simulink model "provablock"  (Simulink 7.4)
settings: Solver=ode45  StartTime=0.0  StopTime=10.0  RelTol=1e-3
values from neighbouring files (symbols this model uses):
  robot = wam    [WAMforcecontrol.m]    (also in batchwamobs.m; controltest.m; feedforward.m; inertia2.m = p560)
undefined symbols (not defined in the file or in its folder): selectde, selectdx1e, selectdx2e
settings Model: Creator=acolome  LastModifiedBy=acolome

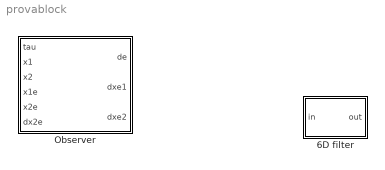
== system provablock ==
  6D filter : Subsystem  mask{K=1, tau=6*pi}
      mask prompts: K "Gain"; tau "time constant"
  Observer : Subsystem  mask{robot=robot, g=[0 0 9.81]}
      mask prompts: robot "Robot Object"; g "Gravity"
      mask Display:
      | port_label('output',1,'de')
      | port_label('output', 2, 'dxe1')
      | port_label('output', 3, 'dxe2')
      | 
      | port_label('input', 1, 'tau')
      | port_label('input', 2, 'q')
      | port_label('input', 3, 'dq')
      | port_label('input', 4, 'x1e')
      | port_label('input', 5, 'x2e')
      | port_label('input', 6, 'dx2e')

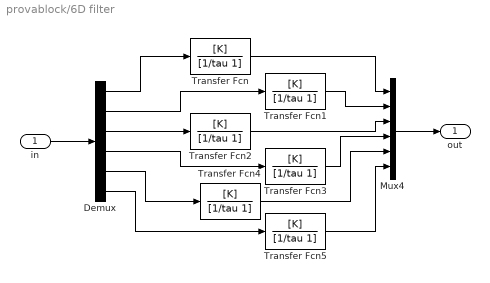
== system provablock/6D filter ==
  in : Inport  OutDataType=fixdt(1, 16)  OutScaling=2^0
  Demux : Demux  Outputs=6
  Mux4 : Mux  Inputs=6
  Transfer Fcn{,1..5} (6 alike) : TransferFcn  Numerator=[K]  Denominator=[1/tau 1]
  out : Outport  OutDataType=fixdt(1, 16)  OutScaling=2^0
  wires:
  Demux/1 -> Transfer Fcn/1
  Demux/2 -> Transfer Fcn1/1
  Demux/3 -> Transfer Fcn2/1
  Demux/4 -> Transfer Fcn3/1
  Demux/5 -> Transfer Fcn4/1
  Demux/6 -> Transfer Fcn5/1
  Transfer Fcn/1 -> Mux4/1
  Transfer Fcn1/1 -> Mux4/2
  Transfer Fcn2/1 -> Mux4/3
  Transfer Fcn3/1 -> Mux4/4
  Transfer Fcn4/1 -> Mux4/5
  Transfer Fcn5/1 -> Mux4/6
  Mux4/1 -> out/1
  in/1 -> Demux/1

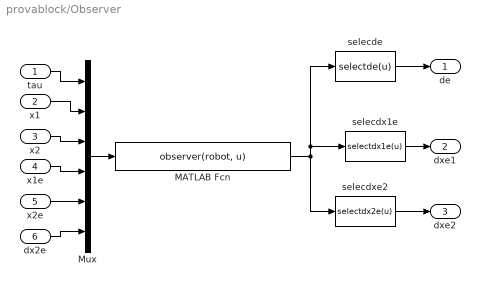
== system provablock/Observer ==
  tau : Inport  OutDataType=fixdt(1, 16)  OutScaling=2^0
  x1 : Inport  Port=2  OutDataType=fixdt(1, 16)  OutScaling=2^0
  x2 : Inport  Port=3  OutDataType=fixdt(1, 16)  OutScaling=2^0
  x1e : Inport  Port=4  OutDataType=fixdt(1, 16)  OutScaling=2^0
  x2e : Inport  Port=5  OutDataType=fixdt(1, 16)  OutScaling=2^0
  dx2e : Inport  Port=6  OutDataType=fixdt(1, 16)  OutScaling=2^0
  MATLAB Fcn : MATLABFcn  MATLABFcn=observer(robot, u)  OutputDimensions=n
  Mux : Mux  Inputs=6
  selecde : MATLABFcn  MATLABFcn=selectde(u)
  selecdx1e : MATLABFcn  MATLABFcn=selectdx1e(u)
  selecdxe2 : MATLABFcn  MATLABFcn=selectdx2e(u)
  de : Outport  OutDataType=fixdt(1, 16)  OutScaling=2^0
  dxe1 : Outport  Port=2  OutDataType=fixdt(1, 16)  OutScaling=2^0
  dxe2 : Outport  Port=3  OutDataType=fixdt(1, 16)  OutScaling=2^0
  wires:
  Mux/1 -> MATLAB Fcn/1
  tau/1 -> Mux/1
  x1/1 -> Mux/2
  x2/1 -> Mux/3
  x1e/1 -> Mux/4
  x2e/1 -> Mux/5
  dx2e/1 -> Mux/6
  MATLAB Fcn/1 -> selecde/1, selecdx1e/1, selecdxe2/1
  selecde/1 -> de/1
  selecdx1e/1 -> dxe1/1
  selecdxe2/1 -> dxe2/1
